simulink model "adrc1"  (Simulink 6.0)
settings: Solver=ode3  StartTime=0.0  StopTime=60  FixedStep=0.1  RelTol=1e-3
settings Model: LastModifiedBy=dell
settings OptimizationCC: InlineInvariantSignals=off
settings DebuggingCC: AlgebraicLoopMsg=none  SolverPrmCheckMsg=none

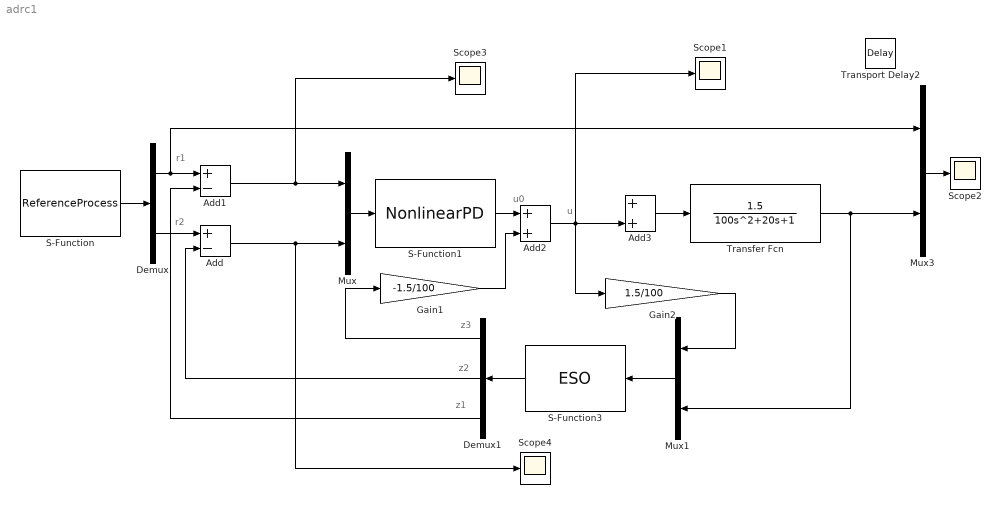
== system adrc1 ==
  note: u0
  note: z3
  note: z2
  note: z1
  note: r1
  note: r2
  note: u
  Add : Sum  Inputs=+-  OutScaling=2^-10
  Add1 : Sum  Inputs=+-  OutScaling=2^-10
  Add2 : Sum  OutScaling=2^-10
  Add3 : Sum  OutScaling=2^-10
  Demux : Demux  Outputs=2
  Demux1 : Demux  Orientation=left  Outputs=3
  Gain1 : Gain  Gain=-1.5/100
  Gain2 : Gain  Gain=1.5/100
  Mux : Mux  Inputs=2
  Mux1 : Mux  Orientation=left  Inputs=2
  Mux3 : Mux  Inputs=2
  S-Function : S-Function  FunctionName=ReferenceProcess  Parameters=SetPoint, RisingTime,SampleTime  mask{SetPoint=1, RisingTime=8, SampleTime=0.1}
  S-Function1 : S-Function  FunctionName=NonlinearPD  Parameters=Beta1,Beta2,Delta,A1,A2,SampleTime  mask{Beta1=150, Beta2=100, Delta=0.2, A1=3/4, A2=3/2, SampleTime=0.1}
      mask prompts: Beta1 "Proportion Coefficient"; Beta2 "Derivation Coefficient"; Delta "Linear Region"; A1 "Proportion Power"; A2 "Derivation Power"; SampleTime "Sample Time"
  S-Function3 : S-Function  Orientation=left  FunctionName=ESO  Parameters=SampleTime,Delta,Beta1,Beta2,Beta3  mask{Delta=0.1, Beta1=20, Beta2=25, Beta3=30, SampleTime=0.1}
      mask prompts: Delta "Linear Region"; Beta1 "Observer Coefficient 1"; Beta2 "Observer Coefficient 2"; Beta3 "Observer Coefficient 3"; SampleTime "Sample Time"
  Scope{1..4} (4 alike) : Scope
      Scope1 settings: TimeRange=3.16679535927733e-007  YMin=0.996252  YMax=0.99644
      Scope2 settings: TimeRange=16.01890756302521  YMin=0  YMax=1.28157  SaveName=ScopeData10
      Scope3 settings: TimeRange=3.16679535927733e-007  YMin=0.9962515155865817  YMax=0.9964397232263716
      Scope4 settings: TimeRange=3.16679535927733e-007  YMin=0.996252  YMax=0.99644  SaveName=ScopeData2
  Transfer Fcn : TransferFcn  Numerator=1.5  Denominator="[100 20  1]"
  Transport Delay2 : TransportDelay  DelayTime=0.2
  wires:
  S-Function/1 -> Demux/1
  Demux/2 -> Add/1
  Demux/1 -> Add1/1, Mux3/1
  S-Function3/1 -> Demux1/1
  Demux1/3 -> Add1/2
  Demux1/2 -> Add/2
  Add1/1 -> Mux/1, Scope3/1
  Add/1 -> Mux/2, Scope4/1
  Mux/1 -> S-Function1/1
  Add2/1 -> Gain2/1, Add3/2, Scope1/1
  Transfer Fcn/1 -> Mux1/2, Mux3/2
  Mux1/1 -> S-Function3/1
  Demux1/1 -> Gain1/1
  Gain1/1 -> Add2/2
  S-Function1/1 -> Add2/1
  Gain2/1 -> Mux1/1
  Mux3/1 -> Scope2/1
  Add3/1 -> Transfer Fcn/1
